simulink model "simulink_PDI"  (R2025b)
settings: Solver=ode23  StartTime=0.0  StopTime=10  RelTol=1e-3
values from neighbouring files (symbols this model uses):
  alpha_0 = invpendulumP.alpha_0    [CODE_42_01.m]    (also in nonlinear_analisys_and_simulation.m)
  alpha_1 = invpendulumP.alpha_1    [CODE_42_01.m]    (also in nonlinear_analisys_and_simulation.m)
  b = invpendulumP.b    [CODE_42_01.m]    (also in nonlinear_analisys_and_simulation.m)
  c = invpendulumP.c    [CODE_42_01.m]    (also in nonlinear_analisys_and_simulation.m)
  g = invpendulumP.g    [CODE_42_01.m]    (also in nonlinear_analisys_and_simulation.m)
  I_0 = invpendulumP.I_0    [CODE_42_01.m]    (also in nonlinear_analisys_and_simulation.m)
  I_1 = invpendulumP.I_1    [CODE_42_01.m]    (also in nonlinear_analisys_and_simulation.m)
  I_2 = invpendulumP.I_2    [CODE_42_01.m]    (also in nonlinear_analisys_and_simulation.m)
  kd = 1    [CODE_42_01.m]    (also in nonlinear_analisys_and_simulation.m)
  ki = 2    [CODE_42_01.m]    (also in nonlinear_analisys_and_simulation.m)
  kp = 8    [CODE_42_01.m]    (also in nonlinear_analisys_and_simulation.m)
  kt = invpendulumP.kt    [CODE_42_01.m]    (also in nonlinear_analisys_and_simulation.m)
  M = invpendulumP.M    [CODE_42_01.m]    (also in nonlinear_analisys_and_simulation.m)
  r = invpendulumP.r    [CODE_42_01.m]    (also in nonlinear_analisys_and_simulation.m)
settings Model: Creator=massi  LastModifiedBy=palla

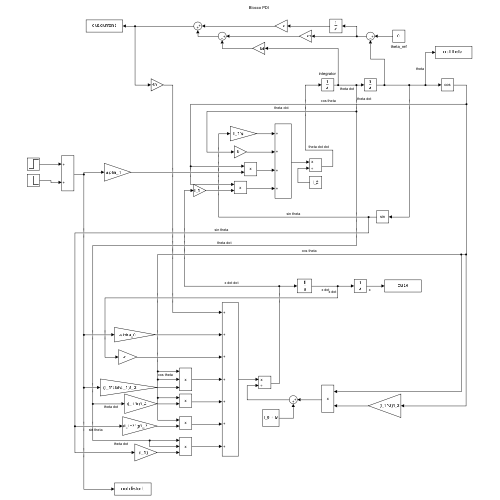
[thumbnail: Simulink's stored preview of the top-level diagram]
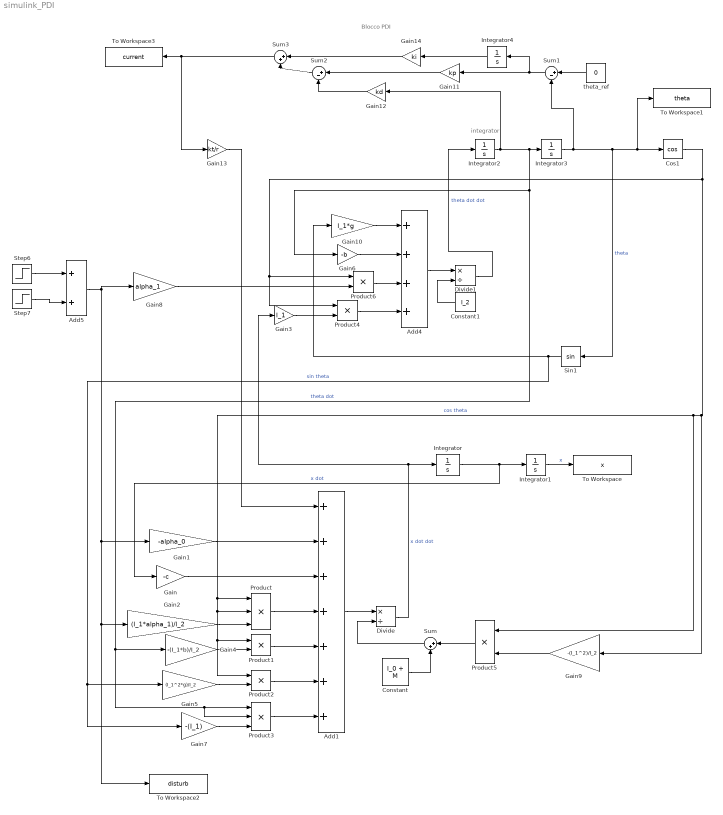
== system simulink_PDI ==
  note: Blocco PDI
  note: integrator
  Add1 : Sum  Inputs=+++++++
  Add4 : Sum  Inputs=++++
  Add5 : Sum
  Constant : Constant  Value=I_0 + M
  Constant1 : Constant  Value=I_2
  Cos1 : Trigonometry  Operator=cos
  Divide : Product  Inputs=*/
  Divide1 : Product  Inputs=*/
  Gain : Gain  Gain=-c
  Gain1 : Gain  Gain=-alpha_0
  Gain10 : Gain  Gain=I_1*g
  Gain11 : Gain  Gain=kp
  Gain12 : Gain  Gain=kd
  Gain13 : Gain  Gain=kt/r
  Gain14 : Gain  Gain=ki
  Gain2 : Gain  Gain=(I_1*alpha_1)/I_2
  Gain3 : Gain  Gain=I_1
  Gain4 : Gain  Gain=-(I_1*b)/I_2
  Gain5 : Gain  Gain=(I_1^2*g)/I_2
  Gain6 : Gain  Gain=-b
  Gain7 : Gain  Gain=-(I_1)
  Gain8 : Gain  Gain=alpha_1
  Gain9 : Gain  Gain=-(I_1^2)/I_2
  Integrator{,1..4} (5 alike) : Integrator
  Product : Product  Inputs=3
  Product{1..2,4..6} (5 alike) : Product
  Product3 : Product  Inputs=3
  Sin1 : Trigonometry
  Step6 : Step  SampleTime=0
  Step7 : Step  Time=3  After=-1  SampleTime=0
  Sum : Sum  Inputs=|++
  Sum1 : Sum  Inputs=|+-
  Sum2 : Sum  Inputs=|+-
  Sum3 : Sum  Inputs=|++
  To Workspace : ToWorkspace  VariableName=x  SampleTime=-1
  To Workspace1 : ToWorkspace  VariableName=theta  SampleTime=-1
  To Workspace2 : ToWorkspace  VariableName=disturb  SaveFormat=Timeseries  SampleTime=-1
  To Workspace3 : ToWorkspace  VariableName=current  SampleTime=-1
  theta_ref : Constant  Value=0
  wires:
  Gain8/1 -> Product6/2
  Step7/1 -> Add5/2
  Integrator1/1 -> To Workspace/1  "x"
  Cos1/1 -> Product/1, Product/2, Product1/1, Product2/1, Product5/1, Gain9/1, Product6/1, Product4/1  "cos theta"
  Constant1/1 -> Divide1/2
  Integrator2/1 -> Gain12/1, Gain6/1, Gain4/1, Product3/2, Product3/1, Integrator3/1  "theta dot"
  Sum1/1 -> Integrator4/1, Gain11/1
  Add4/1 -> Divide1/1
  Gain9/1 -> Product5/2
  Integrator/1 -> Gain/1, Integrator1/1  "x dot"
  Sin1/1 -> Gain10/1, Gain5/1, Gain7/1  "sin theta"
  Gain2/1 -> Product/3
  Gain1/1 -> Add1/2
  theta_ref/1 -> Sum1/1
  Product2/1 -> Add1/6
  Product4/1 -> Add4/4
  Sum2/1 -> Sum3/2
  Gain5/1 -> Product2/2
  Gain/1 -> Add1/3
  Gain6/1 -> Add4/2
  Gain4/1 -> Product1/2
  Product5/1 -> Sum/1
  Constant/1 -> Sum/2
  Product6/1 -> Add4/3
  Add5/1 -> Gain8/1, Gain2/1, To Workspace2/1, Gain1/1
  Sum/1 -> Divide/2
  Gain10/1 -> Add4/1
  Product3/1 -> Add1/7
  Integrator3/1 -> To Workspace1/1, Cos1/1, Sin1/1, Sum1/2  "theta"
  Gain11/1 -> Sum2/1
  Divide/1 -> Gain3/1, Integrator/1  "x dot dot"
  Step6/1 -> Add5/1
  Product1/1 -> Add1/5
  Divide1/1 -> Integrator2/1  "theta dot dot"
  Add1/1 -> Divide/1
  Gain13/1 -> Add1/1
  Gain7/1 -> Product3/3
  Gain12/1 -> Sum2/2
  Gain3/1 -> Product4/2
  Product/1 -> Add1/4
  Integrator4/1 -> Gain14/1
  Gain14/1 -> Sum3/1
  Sum3/1 -> Gain13/1, To Workspace3/1
